simulink model "lab_1"  (R2016a)
settings: Solver=VariableStepAuto  SolverMode=SingleTasking  StartTime=0.0  StopTime=50  RelTol=1e-3
settings Model: Creator=Универская хуета  LastModifiedBy=Универская хуета
settings DataIOCC: LimitDataPoints=on  SaveOutput=off  SaveTime=off
settings OptimizationCC: BlockReduction=off  BooleanDataType=off
settings DebuggingCC: SaveWithParameterizedLinksMsg=none  UnderspecifiedInitializationDetection=Classic  MergeDetectMultiDrivingBlocksExec=none  SignalResolutionControl=TryResolveAllWithWarning  AllowSymbolicDim=off
settings HardwareCC: TargetUnknown=on

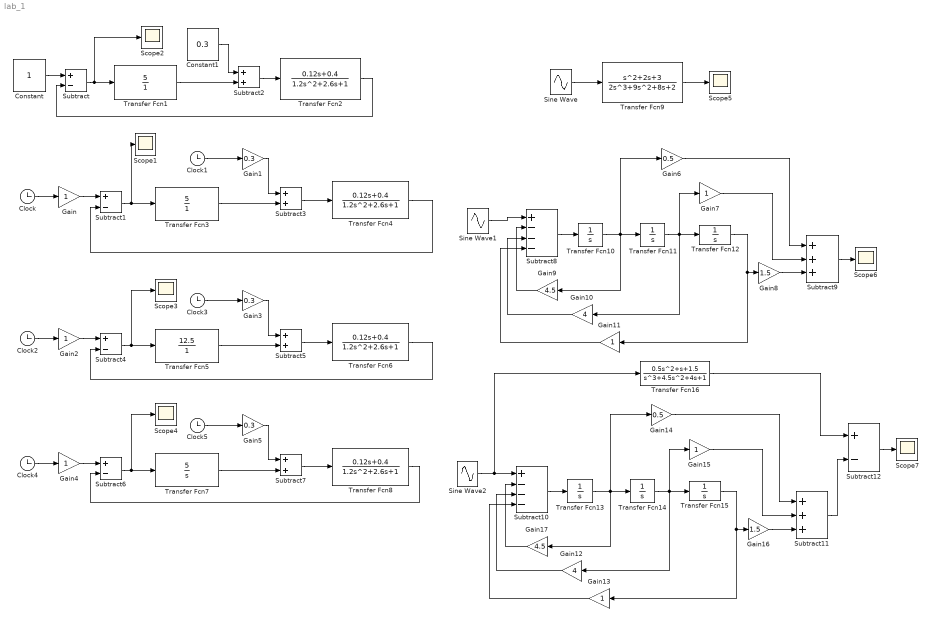
== system lab_1 ==
  Clock{,1..5} (6 alike) : Clock
  Constant : Constant
  Constant1 : Constant  Value=0.3
  Gain{,2,4,7,11,13,15} (7 alike) : Gain
  Gain1 : Gain  Gain=0.3
  Gain10 : Gain  Gain=4
  Gain12 : Gain  Gain=4
  Gain14 : Gain  Gain=0.5
  Gain16 : Gain  Gain=1.5
  Gain17 : Gain  Gain=4.5
  Gain3 : Gain  Gain=0.3
  Gain5 : Gain  Gain=0.3
  Gain6 : Gain  Gain=0.5
  Gain8 : Gain  Gain=1.5
  Gain9 : Gain  Gain=4.5
  Scope{1..7} (7 alike) : Scope
  Sine Wave : Sin  SampleTime=0
  Sine Wave1 : Sin  SampleTime=0
  Sine Wave2 : Sin  SampleTime=0
  Subtract{,1,4,6,12} (5 alike) : Sum  Inputs=+-
  Subtract10 : Sum  Inputs=+---
  Subtract11 : Sum  Inputs=+++
  Subtract{2..3,5,7} (4 alike) : Sum
  Subtract8 : Sum  Inputs=+---
  Subtract9 : Sum  Inputs=+++
  Transfer Fcn1 : TransferFcn  Numerator=[5]  Denominator=[1]
  Transfer Fcn{10..15} (6 alike) : TransferFcn  Denominator=[1 0]
  Transfer Fcn16 : TransferFcn  Numerator=[0.5 1 1.5]  Denominator=[1 4.5 4 1]
  Transfer Fcn{2,4,6,8} (4 alike) : TransferFcn  Numerator=[0.12 0.4]  Denominator=[1.2 2.6 1]
  Transfer Fcn3 : TransferFcn  Numerator=[5]  Denominator=[1]
  Transfer Fcn5 : TransferFcn  Numerator=[12.5]  Denominator=[1]
  Transfer Fcn7 : TransferFcn  Numerator=5  Denominator=[1 0]
  Transfer Fcn9 : TransferFcn  Numerator=[1 2 3]  Denominator=[2 9 8 2]
  wires:
  Constant/1 -> Subtract/1
  Transfer Fcn1/1 -> Subtract2/2
  Transfer Fcn2/1 -> Subtract/2
  Constant1/1 -> Subtract2/1
  Subtract/1 -> Transfer Fcn1/1, Scope2/1
  Transfer Fcn3/1 -> Subtract3/2
  Transfer Fcn4/1 -> Subtract1/2
  Subtract1/1 -> Transfer Fcn3/1, Scope1/1
  Gain/1 -> Subtract1/1
  Clock/1 -> Gain/1
  Clock1/1 -> Gain1/1
  Gain1/1 -> Subtract3/1
  Subtract2/1 -> Transfer Fcn2/1
  Subtract3/1 -> Transfer Fcn4/1
  Transfer Fcn5/1 -> Subtract5/2
  Transfer Fcn6/1 -> Subtract4/2
  Subtract4/1 -> Transfer Fcn5/1, Scope3/1
  Gain2/1 -> Subtract4/1
  Clock2/1 -> Gain2/1
  Clock3/1 -> Gain3/1
  Gain3/1 -> Subtract5/1
  Subtract5/1 -> Transfer Fcn6/1
  Transfer Fcn7/1 -> Subtract7/2
  Transfer Fcn8/1 -> Subtract6/2
  Subtract6/1 -> Transfer Fcn7/1, Scope4/1
  Gain4/1 -> Subtract6/1
  Clock4/1 -> Gain4/1
  Clock5/1 -> Gain5/1
  Gain5/1 -> Subtract7/1
  Subtract7/1 -> Transfer Fcn8/1
  Sine Wave/1 -> Transfer Fcn9/1
  Transfer Fcn9/1 -> Scope5/1
  Sine Wave1/1 -> Subtract8/1
  Transfer Fcn11/1 -> Gain7/1, Gain10/1, Transfer Fcn12/1
  Transfer Fcn10/1 -> Gain9/1, Gain6/1, Transfer Fcn11/1
  Subtract8/1 -> Transfer Fcn10/1
  Transfer Fcn12/1 -> Gain11/1, Gain8/1
  Gain9/1 -> Subtract8/2
  Gain10/1 -> Subtract8/3
  Gain11/1 -> Subtract8/4
  Gain6/1 -> Subtract9/1
  Gain7/1 -> Subtract9/2
  Gain8/1 -> Subtract9/3
  Subtract9/1 -> Scope6/1
  Sine Wave2/1 -> Subtract10/1, Transfer Fcn16/1
  Transfer Fcn14/1 -> Gain15/1, Gain12/1, Transfer Fcn15/1
  Transfer Fcn13/1 -> Gain17/1, Gain14/1, Transfer Fcn14/1
  Subtract10/1 -> Transfer Fcn13/1
  Transfer Fcn15/1 -> Gain13/1, Gain16/1
  Gain17/1 -> Subtract10/2
  Gain12/1 -> Subtract10/3
  Gain13/1 -> Subtract10/4
  Gain14/1 -> Subtract11/1
  Gain15/1 -> Subtract11/2
  Gain16/1 -> Subtract11/3
  Subtract12/1 -> Scope7/1
  Transfer Fcn16/1 -> Subtract12/1
  Subtract11/1 -> Subtract12/2
